simulink model "PTC_MBDS_SetBit_Sample"  (R2013a)
settings: Solver=FixedStepDiscrete  StartTime=0.0  StopTime=100  FixedStep=Auto  RelTol=1e-3
libraries: simulink x12, PTC_MBDS_LIB x4, simulink_extras x1
settings Model: Creator=uidl7367  LastModifiedBy=sundeep.tuteja
settings DataIOCC: SignalLoggingSaveFormat=ModelDataLogs
settings OptimizationCC: ExpressionDepthLimit=2147483647  InitFltsAndDblsToZero=on
settings DebuggingCC: SaveWithParameterizedLinksMsg=none  SignalResolutionControl=TryResolveAllWithWarning  SolverPrmCheckMsg=none  InheritedTsInSrcMsg=none  MultiTaskDSMMsg=warning  MultiTaskCondExecSysMsg=none  FcnCallInpInsideContextMsg=UseLocalSettings  StrictBusMsg=Warning
settings RTWCC: IncludeERTFirstTime=on
settings GRTTargetCC: TargetFcnLib=ansi_tfl_tmw.mat  CombineOutputUpdateFcns=off  GRTInterface=on

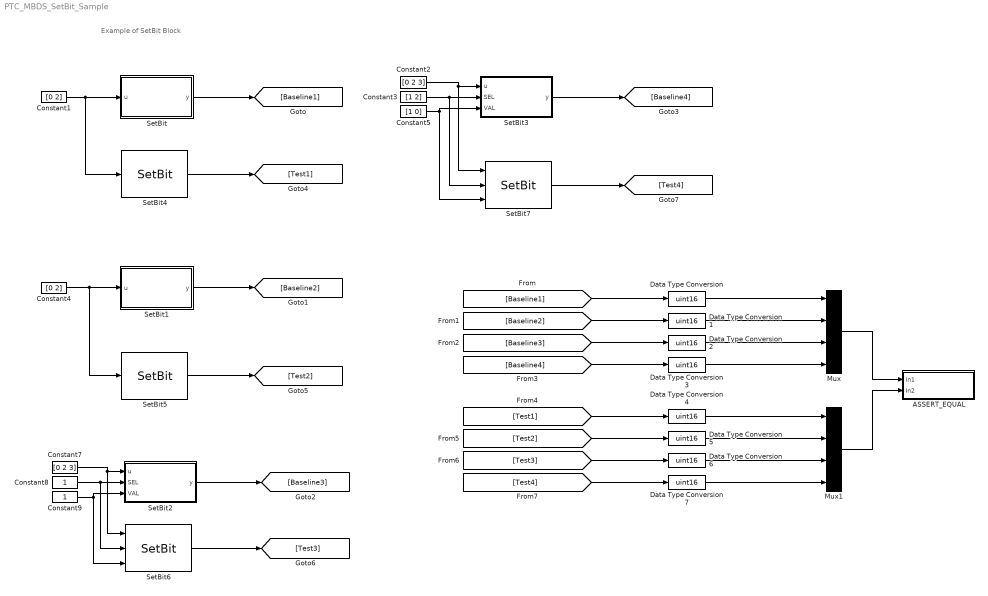
== system PTC_MBDS_SetBit_Sample ==
  note: Example of SetBit Block
  ASSERT_EQUAL : Subsystem
  Constant1 : Constant  InitFcn=|  Value=[0 2]  VectorParams1D=off  OutDataTypeStr=uint8
      | if(exist('MBDS_BlockCallback', 'file'))
      |    MBDS_BlockCallback('Update', gcb);  
      | end
  Constant2 : Constant  InitFcn=|  Value=[0 2 3]  VectorParams1D=off  OutDataTypeStr=uint16
      | if(exist('MBDS_BlockCallback', 'file'))
      |    MBDS_BlockCallback('Update', gcb);  
      | end
  Constant3 : Constant  InitFcn=|  Value=[1 2]  VectorParams1D=off  OutDataTypeStr=uint8
      | if(exist('MBDS_BlockCallback', 'file'))
      |    MBDS_BlockCallback('Update', gcb);  
      | end
  Constant4 : Constant  InitFcn=|  Value=[0 2]  VectorParams1D=off  OutDataTypeStr=uint8
      | if(exist('MBDS_BlockCallback', 'file'))
      |    MBDS_BlockCallback('Update', gcb);  
      | end
  Constant5 : Constant  InitFcn=|  Value=[1 0]  VectorParams1D=off  OutDataTypeStr=boolean
      | if(exist('MBDS_BlockCallback', 'file'))
      |    MBDS_BlockCallback('Update', gcb);  
      | end
  Constant7 : Constant  InitFcn=|  Value=[0 2 3]  VectorParams1D=off  OutDataTypeStr=uint16
      | if(exist('MBDS_BlockCallback', 'file'))
      |    MBDS_BlockCallback('Update', gcb);  
      | end
  Constant8 : Constant  InitFcn=|  VectorParams1D=off  OutDataTypeStr=uint8
      | if(exist('MBDS_BlockCallback', 'file'))
      |    MBDS_BlockCallback('Update', gcb);  
      | end
  Constant9 : Constant  InitFcn=|  VectorParams1D=off  OutDataTypeStr=boolean
      | if(exist('MBDS_BlockCallback', 'file'))
      |    MBDS_BlockCallback('Update', gcb);  
      | end
  Data Type Conversion{,1..7} (8 alike) : DataTypeConversion  OutDataTypeStr=uint16
  Mux : Mux
  Mux1 : Mux
  SetBit : Subsystem  InitFcn=|  mask(SetBit){MBDS_LibraryBlock=on, ZeroIndexing=off, SEL_Enabled=off, SEL=1, VAL_Enabled=off, VAL=1, MBDS_BlockVersion=05.40}
      | if(exist('MBDS_BlockCallback', 'file'))
      |    MBDS_BlockCallback('Update', gcb);
      | end
      mask prompts: MBDS_LibraryBlock "MBDS library block"; ZeroIndexing "Use zero-based indexing"; SEL_Enabled "Show SEL port"; SEL "Bit selection:"; VAL_Enabled "Show VAL port"; VAL "Bit value:"; MBDS_BlockVersion "Block version:"
      mask help: Set or reset specified bits of a input signal.
      mask init:
      | if(exist('MBDS_BlockCallback', 'file'))
      |    MBDS_BlockCallback('Init', gcb);
      | else
      |    % Disable all mask parameters
      |    MaskEnables = get_param(gcb, 'MaskEnables');
      |    for k = [1:length(MaskEnables)]
      |       MaskEnables{k} = 'off';
      |    end
      |    if(~isequal(MaskEnables, get_param(gcb, 'MaskEnables')))
      |       set_param(gcb, 'MaskEnables', MaskEnables);
      |    end
      | end
      settings: AttributesFormatString=|
      | Zero-based indexing: %<ZeroIndexing>
      | VAL = %<VAL>
      mask Help: eval(['open([workdir(''library_dir:''),''\Blockset\help\'',get_param(gcb,''MaskType''),''.html''])'])
      mask Callback ZeroIndexing:
      | % Adopt Value
      | if(exist('MBDS_BlockCallback', 'file'))
      |    MBDS_BlockCallback('ZeroIndexing', gcb);
      | end
      mask Callback SEL_Enabled:
      | % Update mask parameter dialog
      | if(exist('MBDS_BlockCallback', 'file'))
      |    MBDS_BlockCallback('SEL_Enabled', gcb);
      | end
      mask Callback SEL:
      | % Adopt Value
      | if(exist('MBDS_BlockCallback', 'file'))
      |    MBDS_BlockCallback('SEL', gcb);
      | end
      mask Callback VAL_Enabled:
      | % Update mask parameter dialog
      | if(exist('MBDS_BlockCallback', 'file'))
      |    MBDS_BlockCallback('VAL_Enabled', gcb);
      | end
      mask Callback VAL:
      | % Adopt Value
      | if(exist('MBDS_BlockCallback', 'file'))
      |    MBDS_BlockCallback('VAL', gcb);
      | end
      mask Display:
      | % Show block text
      | disp(sprintf('Set Bit'));
      | 
      | % Display port labels
      | port_label('input', 1, 'u');
      | port_label('output', 1, 'y');
  SetBit1 : Subsystem  InitFcn=|  mask(SetBit){MBDS_LibraryBlock=on, ZeroIndexing=on, SEL_Enabled=off, SEL=0, VAL_Enabled=off, VAL=1, MBDS_BlockVersion=05.40}
      | if(exist('MBDS_BlockCallback', 'file'))
      |    MBDS_BlockCallback('Update', gcb);
      | end
      mask prompts: MBDS_LibraryBlock "MBDS library block"; ZeroIndexing "Use zero-based indexing"; SEL_Enabled "Show SEL port"; SEL "Bit selection:"; VAL_Enabled "Show VAL port"; VAL "Bit value:"; MBDS_BlockVersion "Block version:"
      mask help: Set or reset specified bits of a input signal.
      mask init: same as PTC_MBDS_SetBit_Sample/SetBit
      settings: AttributesFormatString=|
      | Zero-based indexing: %<ZeroIndexing>
      | VAL = %<VAL>
      mask Help: eval(['open([workdir(''library_dir:''),''\Blockset\help\'',get_param(gcb,''MaskType''),''.html''])'])
      mask Callback ZeroIndexing:
      | % Adopt Value
      | if(exist('MBDS_BlockCallback', 'file'))
      |    MBDS_BlockCallback('ZeroIndexing', gcb);
      | end
      mask Callback SEL_Enabled:
      | % Update mask parameter dialog
      | if(exist('MBDS_BlockCallback', 'file'))
      |    MBDS_BlockCallback('SEL_Enabled', gcb);
      | end
      mask Callback SEL:
      | % Adopt Value
      | if(exist('MBDS_BlockCallback', 'file'))
      |    MBDS_BlockCallback('SEL', gcb);
      | end
      mask Callback VAL_Enabled:
      | % Update mask parameter dialog
      | if(exist('MBDS_BlockCallback', 'file'))
      |    MBDS_BlockCallback('VAL_Enabled', gcb);
      | end
      mask Callback VAL:
      | % Adopt Value
      | if(exist('MBDS_BlockCallback', 'file'))
      |    MBDS_BlockCallback('VAL', gcb);
      | end
      mask Display:
      | % Show block text
      | disp(sprintf('Set Bit'));
      | 
      | % Display port labels
      | port_label('input', 1, 'u');
      | port_label('output', 1, 'y');
  SetBit2 : Subsystem  InitFcn=|  mask(SetBit){MBDS_LibraryBlock=on, ZeroIndexing=off, SEL_Enabled=on, SEL=0, VAL_Enabled=on, VAL=0, MBDS_BlockVersion=05.40}
      | if(exist('MBDS_BlockCallback', 'file'))
      |    MBDS_BlockCallback('Update', gcb);
      | end
      mask prompts: MBDS_LibraryBlock "MBDS library block"; ZeroIndexing "Use zero-based indexing"; SEL_Enabled "Show SEL port"; SEL "Bit selection:"; VAL_Enabled "Show VAL port"; VAL "Bit value:"; MBDS_BlockVersion "Block version:"
      mask help: Set or reset specified bits of a input signal.
      mask init: same as PTC_MBDS_SetBit_Sample/SetBit
      settings: AttributesFormatString=Zero-based indexing: %<ZeroIndexing>
      mask Help: eval(['open([workdir(''library_dir:''),''\Blockset\help\'',get_param(gcb,''MaskType''),''.html''])'])
      mask Callback ZeroIndexing:
      | % Adopt Value
      | if(exist('MBDS_BlockCallback', 'file'))
      |    MBDS_BlockCallback('ZeroIndexing', gcb);
      | end
      mask Callback SEL_Enabled:
      | % Update mask parameter dialog
      | if(exist('MBDS_BlockCallback', 'file'))
      |    MBDS_BlockCallback('SEL_Enabled', gcb);
      | end
      mask Callback SEL:
      | % Adopt Value
      | if(exist('MBDS_BlockCallback', 'file'))
      |    MBDS_BlockCallback('SEL', gcb);
      | end
      mask Callback VAL_Enabled:
      | % Update mask parameter dialog
      | if(exist('MBDS_BlockCallback', 'file'))
      |    MBDS_BlockCallback('VAL_Enabled', gcb);
      | end
      mask Callback VAL:
      | % Adopt Value
      | if(exist('MBDS_BlockCallback', 'file'))
      |    MBDS_BlockCallback('VAL', gcb);
      | end
      mask Display:
      | % Show block text
      | disp(sprintf('Set Bit'));
      | 
      | % Display port labels
      | port_label('input', 1, 'u');
      | port_label('input', 2, 'SEL');
      | port_label('input', 3, 'VAL');
      | port_label('output', 1, 'y');
  SetBit3 : Subsystem  InitFcn=|  mask(SetBit){MBDS_LibraryBlock=on, ZeroIndexing=off, SEL_Enabled=on, SEL=0, VAL_Enabled=on, VAL=0, MBDS_BlockVersion=05.40}
      | if(exist('MBDS_BlockCallback', 'file'))
      |    MBDS_BlockCallback('Update', gcb);
      | end
      mask prompts: MBDS_LibraryBlock "MBDS library block"; ZeroIndexing "Use zero-based indexing"; SEL_Enabled "Show SEL port"; SEL "Bit selection:"; VAL_Enabled "Show VAL port"; VAL "Bit value:"; MBDS_BlockVersion "Block version:"
      mask help: Set or reset specified bits of a input signal.
      mask init: same as PTC_MBDS_SetBit_Sample/SetBit
      settings: AttributesFormatString=Zero-based indexing: %<ZeroIndexing>
      mask Help: eval(['open([workdir(''library_dir:''),''\Blockset\help\'',get_param(gcb,''MaskType''),''.html''])'])
      mask Callback ZeroIndexing:
      | % Adopt Value
      | if(exist('MBDS_BlockCallback', 'file'))
      |    MBDS_BlockCallback('ZeroIndexing', gcb);
      | end
      mask Callback SEL_Enabled:
      | % Update mask parameter dialog
      | if(exist('MBDS_BlockCallback', 'file'))
      |    MBDS_BlockCallback('SEL_Enabled', gcb);
      | end
      mask Callback SEL:
      | % Adopt Value
      | if(exist('MBDS_BlockCallback', 'file'))
      |    MBDS_BlockCallback('SEL', gcb);
      | end
      mask Callback VAL_Enabled:
      | % Update mask parameter dialog
      | if(exist('MBDS_BlockCallback', 'file'))
      |    MBDS_BlockCallback('VAL_Enabled', gcb);
      | end
      mask Callback VAL:
      | % Adopt Value
      | if(exist('MBDS_BlockCallback', 'file'))
      |    MBDS_BlockCallback('VAL', gcb);
      | end
      mask Display:
      | % Show block text
      | disp(sprintf('Set Bit'));
      | 
      | % Display port labels
      | port_label('input', 1, 'u');
      | port_label('input', 2, 'SEL');
      | port_label('input', 3, 'VAL');
      | port_label('output', 1, 'y');
  SetBit4 : PTC_MBDS_LIB/MBDS Standard Library/Basic Operations/Logic and Bit Operations/SetBit  ZeroIndexing=off  SEL_Enabled=off  SEL=1  VAL_Enabled=off  VAL=1  PTC_MBDS_BlockVersion=5.32  PTC_BlockType=PTC_MBDS_SetBit
      settings: AttributesFormatString=|
      | SEL = %<SEL>
      | VAL = %<VAL>
      | Zero-based indexing: %<ZeroIndexing>
  SetBit5 : PTC_MBDS_LIB/MBDS Standard Library/Basic Operations/Logic and Bit Operations/SetBit  ZeroIndexing=on  SEL_Enabled=off  SEL=0  VAL_Enabled=off  VAL=1  PTC_MBDS_BlockVersion=5.32  PTC_BlockType=PTC_MBDS_SetBit
      settings: AttributesFormatString=|
      | SEL = %<SEL>
      | VAL = %<VAL>
      | Zero-based indexing: %<ZeroIndexing>
  SetBit6 : PTC_MBDS_LIB/MBDS Standard Library/Basic Operations/Logic and Bit Operations/SetBit  ZeroIndexing=off  SEL_Enabled=on  SEL=0  VAL_Enabled=on  VAL=1  PTC_MBDS_BlockVersion=5.32  PTC_BlockType=PTC_MBDS_SetBit
      settings: AttributesFormatString=Zero-based indexing: %<ZeroIndexing>
  SetBit7 : PTC_MBDS_LIB/MBDS Standard Library/Basic Operations/Logic and Bit Operations/SetBit  ZeroIndexing=off  SEL_Enabled=on  SEL=0  VAL_Enabled=on  VAL=1  PTC_MBDS_BlockVersion=5.32  PTC_BlockType=PTC_MBDS_SetBit
      settings: AttributesFormatString=Zero-based indexing: %<ZeroIndexing>
  wires:
  Constant1/1 -> SetBit/1(u), SetBit4/1
  SetBit/1(y) -> [Baseline1]
  Constant4/1 -> SetBit1/1(u), SetBit5/1
  SetBit1/1(y) -> [Baseline2]
  Constant8/1 -> SetBit2/2(SEL), SetBit6/2
  SetBit2/1(y) -> [Baseline3]
  Constant2/1 -> SetBit3/1(u), SetBit7/1
  Constant3/1 -> SetBit3/2(SEL), SetBit7/2
  Constant5/1 -> SetBit3/3(VAL), SetBit7/3
  SetBit3/1(y) -> [Baseline4]
  Constant7/1 -> SetBit2/1(u), SetBit6/1
  Constant9/1 -> SetBit2/3(VAL), SetBit6/3
  SetBit4/1 -> [Test1]
  SetBit5/1 -> [Test2]
  SetBit6/1 -> [Test3]
  SetBit7/1 -> [Test4]
  [Baseline1] -> Data Type Conversion/1
  [Baseline2] -> Data Type Conversion1/1
  [Baseline4] -> Data Type Conversion3/1
  [Baseline3] -> Data Type Conversion2/1
  [Test3] -> Data Type Conversion6/1
  [Test4] -> Data Type Conversion7/1
  [Test2] -> Data Type Conversion5/1
  [Test1] -> Data Type Conversion4/1
  Mux/1 -> ASSERT_EQUAL/1(In1)
  Mux1/1 -> ASSERT_EQUAL/2(In2)
  Data Type Conversion/1 -> Mux/1
  Data Type Conversion1/1 -> Mux/2
  Data Type Conversion2/1 -> Mux/3
  Data Type Conversion3/1 -> Mux/4
  Data Type Conversion4/1 -> Mux1/1
  Data Type Conversion5/1 -> Mux1/2
  Data Type Conversion6/1 -> Mux1/3
  Data Type Conversion7/1 -> Mux1/4

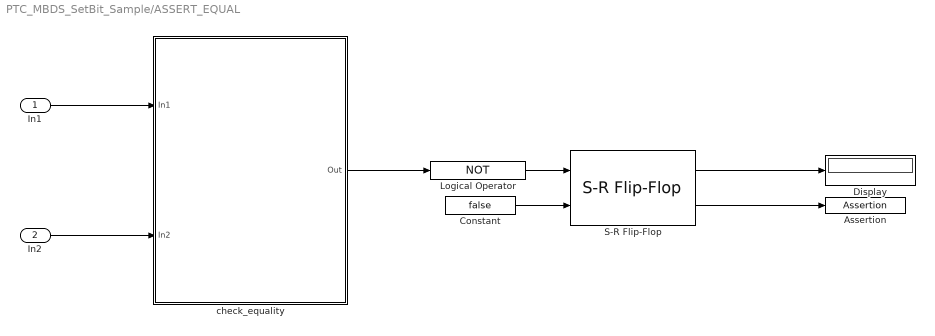
== system PTC_MBDS_SetBit_Sample/ASSERT_EQUAL ==
  In1 : Inport
  In2 : Inport  Port=2
  Assertion : Assertion
  Constant : Constant  Value=false
  Display : Display
  Logical Operator : Logic  Operator=NOT  AllPortsSameDT=off  OutDataTypeStr=boolean
  S-R Flip-Flop : simulink_extras/Flip Flops/S-R Flip-Flop  initial_condition=0
  check_equality : MATLAB Function  TreatAsAtomicUnit=on
  wires:
  S-R Flip-Flop/1 -> Display/1
  check_equality/1(Out) -> Logical Operator/1
  Constant/1 -> S-R Flip-Flop/2
  S-R Flip-Flop/2 -> Assertion/1
  In2/1 -> check_equality/2(In2)
  In1/1 -> check_equality/1(In1)
  Logical Operator/1 -> S-R Flip-Flop/1

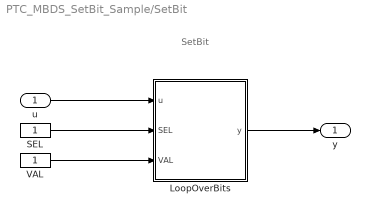
== system PTC_MBDS_SetBit_Sample/SetBit ==
  note: SetBit
  u : Inport
  LoopOverBits : Subsystem
  SEL : Constant  OutDataTypeStr=uint8
  VAL : Constant  OutDataTypeStr=boolean
  y : Outport
  wires:
  LoopOverBits/1(y) -> y/1
  VAL/1 -> LoopOverBits/3(VAL)
  SEL/1 -> LoopOverBits/2(SEL)
  u/1 -> LoopOverBits/1(u)

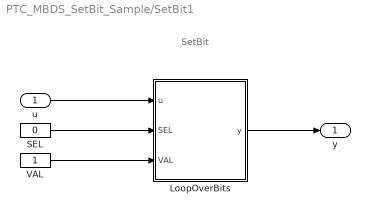
== system PTC_MBDS_SetBit_Sample/SetBit1 ==
  note: SetBit
  u : Inport
  LoopOverBits : Subsystem
  SEL : Constant  Value=0  OutDataTypeStr=uint8
  VAL : Constant  OutDataTypeStr=boolean
  y : Outport
  wires:
  LoopOverBits/1(y) -> y/1
  VAL/1 -> LoopOverBits/3(VAL)
  SEL/1 -> LoopOverBits/2(SEL)
  u/1 -> LoopOverBits/1(u)

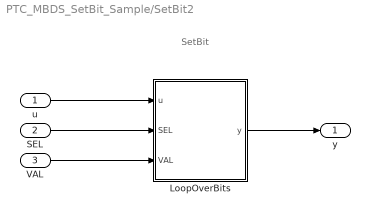
== system PTC_MBDS_SetBit_Sample/SetBit2 ==
  note: SetBit
  u : Inport
  SEL : Inport  Port=2
  VAL : Inport  Port=3  OutDataTypeStr=boolean
  LoopOverBits : Subsystem
  y : Outport
  wires:
  LoopOverBits/1(y) -> y/1
  VAL/1 -> LoopOverBits/3(VAL)
  SEL/1 -> LoopOverBits/2(SEL)
  u/1 -> LoopOverBits/1(u)

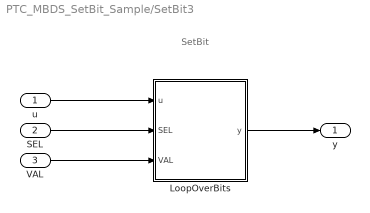
== system PTC_MBDS_SetBit_Sample/SetBit3 ==
  note: SetBit
  u : Inport
  SEL : Inport  Port=2
  VAL : Inport  Port=3  OutDataTypeStr=boolean
  LoopOverBits : Subsystem
  y : Outport
  wires:
  u/1 -> LoopOverBits/1(u)
  SEL/1 -> LoopOverBits/2(SEL)
  VAL/1 -> LoopOverBits/3(VAL)
  LoopOverBits/1(y) -> y/1

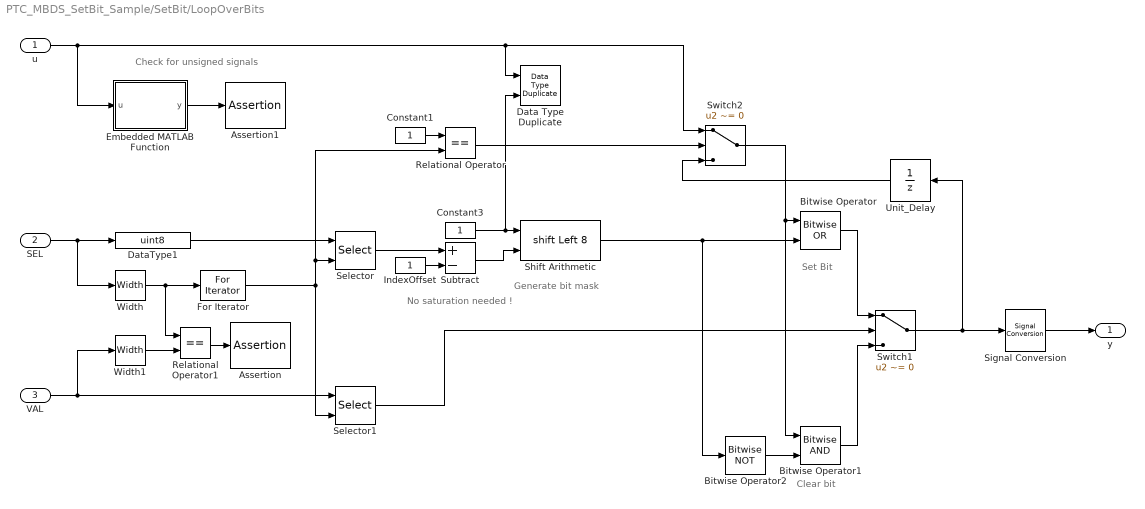
== system PTC_MBDS_SetBit_Sample/SetBit/LoopOverBits ==
  note: No saturation
      | needed !
  note: Generate bit mask
  note: Set Bit
  note: Clear bit
  note: Check for unsigned signals
  u : Inport
  SEL : Inport  Port=2
  VAL : Inport  Port=3
  Assertion : Assertion  AssertionFailFcn=error('Invalid signal dimensions. Bit selection and value specification should have the same dimensions.')
  Assertion1 : Assertion  AssertionFailFcn=error('Invalid data types used for set bit operation. Apply unsigned integer signals only.')
  Bitwise Operator : simulink/Logic and Bit Operations/Bitwise Operator  logicop=OR  UseBitMask=off  NumInputPorts=2  BitMask=bin2dec('11011001')  BitMaskRealWorld=Stored Integer
  Bitwise Operator1 : simulink/Logic and Bit Operations/Bitwise Operator  logicop=AND  UseBitMask=off  NumInputPorts=2  BitMask=bin2dec('11011001')  BitMaskRealWorld=Stored Integer
  Bitwise Operator2 : simulink/Logic and Bit Operations/Bitwise Operator  logicop=NOT  UseBitMask=off  BitMask=bin2dec('11011001')  BitMaskRealWorld=Stored Integer
  Constant1 : Constant  OutDataTypeStr=Inherit: Inherit via back propagation
  Constant3 : Constant  OutDataTypeStr=Inherit: Inherit via back propagation
  Data Type Duplicate : DataTypeDuplicate  InitFcn=|
      | try
      |    MBDS_BlockCallback('Update', gcb);
      | end
  DataType1 : DataTypeConversion  OutDataTypeStr=uint8
  Embedded MATLAB Function : MATLAB Function  TreatAsAtomicUnit=on
  For Iterator : ForIterator  IterationSource=external  IterationVariableDataType=int8
  IndexOffset : Constant  OutDataTypeStr=Inherit: Inherit via back propagation
  Relational Operator : RelationalOperator  Operator===  OutDataTypeStr=boolean
  Relational Operator1 : RelationalOperator  Operator===  OutDataTypeStr=boolean
  Selector : Selector  IndexOptions=Index vector (port)  Indices=[1 3]  OutputSizes=1
  Selector1 : Selector  IndexOptions=Index vector (port)  Indices=[1 3]  OutputSizes=1
  Shift Arithmetic : ArithShift  BitShiftNumberSource=Input port  BitShiftNumber=8  BitShiftDirection=Left
      settings: InputPortMap=u0,p1
  Signal Conversion : SignalConversion
  Subtract : Sum  Inputs=+-  OutDataTypeStr=Inherit: Inherit via back propagation  InputSameDT=on
  Switch1 : Switch  Criteria=u2 ~= 0
  Switch2 : Switch  Criteria=u2 ~= 0
  Unit_Delay : UnitDelay  InitFcn=|  SampleTime=-1
      | try                                  
      |    MBDS_BlockCallback('Update', gcb);
      | end
      settings: AttributesFormatString=Init = %<X0>
  Width : Width  DataType=uint8
  Width1 : Width  DataType=uint8
  y : Outport
  wires:
  Relational Operator1/1 -> Assertion/1
  Width1/1 -> Relational Operator1/2
  Relational Operator/1 -> Switch2/2
  Constant1/1 -> Relational Operator/1
  Unit_Delay/1 -> Switch2/3
  Switch2/1 -> Bitwise Operator1/1, Bitwise Operator/1
  For Iterator/1 -> Selector/2, Relational Operator/2, Selector1/2
  Width/1 -> Relational Operator1/1, For Iterator/1
  Selector1/1 -> Switch1/2
  Shift Arithmetic/1 -> Bitwise Operator2/1, Bitwise Operator/2
  Constant3/1 -> Data Type Duplicate/2, Shift Arithmetic/1
  Switch1/1 -> Signal Conversion/1, Unit_Delay/1
  Bitwise Operator/1 -> Switch1/1
  Bitwise Operator1/1 -> Switch1/3
  Bitwise Operator2/1 -> Bitwise Operator1/2
  Signal Conversion/1 -> y/1
  Subtract/1 -> Shift Arithmetic/2
  Selector/1 -> Subtract/1
  IndexOffset/1 -> Subtract/2
  SEL/1 -> DataType1/1, Width/1
  DataType1/1 -> Selector/1
  VAL/1 -> Selector1/1, Width1/1
  Embedded MATLAB Function/1(y) -> Assertion1/1
  u/1 -> Embedded MATLAB Function/1(u), Data Type Duplicate/1, Switch2/1

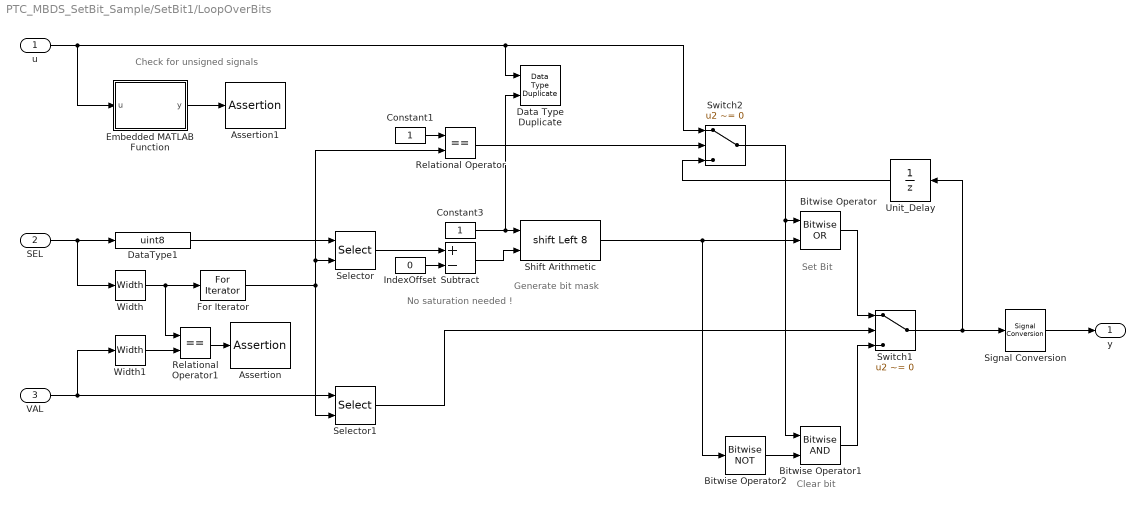
== system PTC_MBDS_SetBit_Sample/SetBit1/LoopOverBits ==
  note: No saturation
      | needed !
  note: Generate bit mask
  note: Set Bit
  note: Clear bit
  note: Check for unsigned signals
  u : Inport
  SEL : Inport  Port=2
  VAL : Inport  Port=3
  Assertion : Assertion  AssertionFailFcn=error('Invalid signal dimensions. Bit selection and value specification should have the same dimensions.')
  Assertion1 : Assertion  AssertionFailFcn=error('Invalid data types used for set bit operation. Apply unsigned integer signals only.')
  Bitwise Operator : simulink/Logic and Bit Operations/Bitwise Operator  logicop=OR  UseBitMask=off  NumInputPorts=2  BitMask=bin2dec('11011001')  BitMaskRealWorld=Stored Integer
  Bitwise Operator1 : simulink/Logic and Bit Operations/Bitwise Operator  logicop=AND  UseBitMask=off  NumInputPorts=2  BitMask=bin2dec('11011001')  BitMaskRealWorld=Stored Integer
  Bitwise Operator2 : simulink/Logic and Bit Operations/Bitwise Operator  logicop=NOT  UseBitMask=off  BitMask=bin2dec('11011001')  BitMaskRealWorld=Stored Integer
  Constant1 : Constant  OutDataTypeStr=Inherit: Inherit via back propagation
  Constant3 : Constant  OutDataTypeStr=Inherit: Inherit via back propagation
  Data Type Duplicate : DataTypeDuplicate  InitFcn=|
      | try
      |    MBDS_BlockCallback('Update', gcb);
      | end
  DataType1 : DataTypeConversion  OutDataTypeStr=uint8
  Embedded MATLAB Function : MATLAB Function  TreatAsAtomicUnit=on
  For Iterator : ForIterator  IterationSource=external  IterationVariableDataType=int8
  IndexOffset : Constant  Value=0  OutDataTypeStr=Inherit: Inherit via back propagation
  Relational Operator : RelationalOperator  Operator===  OutDataTypeStr=boolean
  Relational Operator1 : RelationalOperator  Operator===  OutDataTypeStr=boolean
  Selector : Selector  IndexOptions=Index vector (port)  Indices=[1 3]  OutputSizes=1
  Selector1 : Selector  IndexOptions=Index vector (port)  Indices=[1 3]  OutputSizes=1
  Shift Arithmetic : ArithShift  BitShiftNumberSource=Input port  BitShiftNumber=8  BitShiftDirection=Left
      settings: InputPortMap=u0,p1
  Signal Conversion : SignalConversion
  Subtract : Sum  Inputs=+-  OutDataTypeStr=Inherit: Inherit via back propagation  InputSameDT=on
  Switch1 : Switch  Criteria=u2 ~= 0
  Switch2 : Switch  Criteria=u2 ~= 0
  Unit_Delay : UnitDelay  InitFcn=|  SampleTime=-1
      | try                                  
      |    MBDS_BlockCallback('Update', gcb);
      | end
      settings: AttributesFormatString=Init = %<X0>
  Width : Width  DataType=uint8
  Width1 : Width  DataType=uint8
  y : Outport
  wires:
  Relational Operator1/1 -> Assertion/1
  Width1/1 -> Relational Operator1/2
  Relational Operator/1 -> Switch2/2
  Constant1/1 -> Relational Operator/1
  Unit_Delay/1 -> Switch2/3
  Switch2/1 -> Bitwise Operator1/1, Bitwise Operator/1
  For Iterator/1 -> Selector/2, Relational Operator/2, Selector1/2
  Width/1 -> Relational Operator1/1, For Iterator/1
  Selector1/1 -> Switch1/2
  Shift Arithmetic/1 -> Bitwise Operator2/1, Bitwise Operator/2
  Constant3/1 -> Data Type Duplicate/2, Shift Arithmetic/1
  Switch1/1 -> Signal Conversion/1, Unit_Delay/1
  Bitwise Operator/1 -> Switch1/1
  Bitwise Operator1/1 -> Switch1/3
  Bitwise Operator2/1 -> Bitwise Operator1/2
  Signal Conversion/1 -> y/1
  Subtract/1 -> Shift Arithmetic/2
  Selector/1 -> Subtract/1
  IndexOffset/1 -> Subtract/2
  SEL/1 -> DataType1/1, Width/1
  DataType1/1 -> Selector/1
  VAL/1 -> Selector1/1, Width1/1
  Embedded MATLAB Function/1(y) -> Assertion1/1
  u/1 -> Embedded MATLAB Function/1(u), Data Type Duplicate/1, Switch2/1

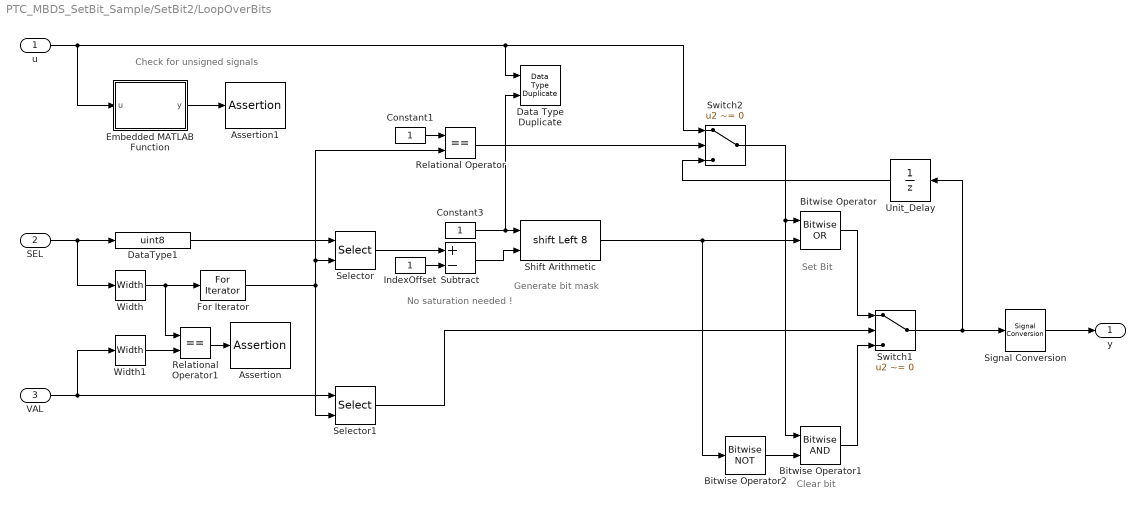
== system PTC_MBDS_SetBit_Sample/SetBit2/LoopOverBits ==
  note: No saturation
      | needed !
  note: Generate bit mask
  note: Set Bit
  note: Clear bit
  note: Check for unsigned signals
  u : Inport
  SEL : Inport  Port=2
  VAL : Inport  Port=3
  Assertion : Assertion  AssertionFailFcn=error('Invalid signal dimensions. Bit selection and value specification should have the same dimensions.')
  Assertion1 : Assertion  AssertionFailFcn=error('Invalid data types used for set bit operation. Apply unsigned integer signals only.')
  Bitwise Operator : simulink/Logic and Bit Operations/Bitwise Operator  logicop=OR  UseBitMask=off  NumInputPorts=2  BitMask=bin2dec('11011001')  BitMaskRealWorld=Stored Integer
  Bitwise Operator1 : simulink/Logic and Bit Operations/Bitwise Operator  logicop=AND  UseBitMask=off  NumInputPorts=2  BitMask=bin2dec('11011001')  BitMaskRealWorld=Stored Integer
  Bitwise Operator2 : simulink/Logic and Bit Operations/Bitwise Operator  logicop=NOT  UseBitMask=off  BitMask=bin2dec('11011001')  BitMaskRealWorld=Stored Integer
  Constant1 : Constant  OutDataTypeStr=Inherit: Inherit via back propagation
  Constant3 : Constant  OutDataTypeStr=Inherit: Inherit via back propagation
  Data Type Duplicate : DataTypeDuplicate  InitFcn=|
      | try
      |    MBDS_BlockCallback('Update', gcb);
      | end
  DataType1 : DataTypeConversion  OutDataTypeStr=uint8
  Embedded MATLAB Function : MATLAB Function  TreatAsAtomicUnit=on
  For Iterator : ForIterator  IterationSource=external  IterationVariableDataType=int8
  IndexOffset : Constant  OutDataTypeStr=Inherit: Inherit via back propagation
  Relational Operator : RelationalOperator  Operator===  OutDataTypeStr=boolean
  Relational Operator1 : RelationalOperator  Operator===  OutDataTypeStr=boolean
  Selector : Selector  IndexOptions=Index vector (port)  Indices=[1 3]  OutputSizes=1
  Selector1 : Selector  IndexOptions=Index vector (port)  Indices=[1 3]  OutputSizes=1
  Shift Arithmetic : ArithShift  BitShiftNumberSource=Input port  BitShiftNumber=8  BitShiftDirection=Left
      settings: InputPortMap=u0,p1
  Signal Conversion : SignalConversion
  Subtract : Sum  Inputs=+-  OutDataTypeStr=Inherit: Inherit via back propagation  InputSameDT=on
  Switch1 : Switch  Criteria=u2 ~= 0
  Switch2 : Switch  Criteria=u2 ~= 0
  Unit_Delay : UnitDelay  InitFcn=|  SampleTime=-1
      | try                                  
      |    MBDS_BlockCallback('Update', gcb);
      | end
      settings: AttributesFormatString=Init = %<X0>
  Width : Width  DataType=uint8
  Width1 : Width  DataType=uint8
  y : Outport
  wires:
  Relational Operator1/1 -> Assertion/1
  Width1/1 -> Relational Operator1/2
  Relational Operator/1 -> Switch2/2
  Constant1/1 -> Relational Operator/1
  Unit_Delay/1 -> Switch2/3
  Switch2/1 -> Bitwise Operator1/1, Bitwise Operator/1
  For Iterator/1 -> Selector/2, Relational Operator/2, Selector1/2
  Width/1 -> Relational Operator1/1, For Iterator/1
  Selector1/1 -> Switch1/2
  Shift Arithmetic/1 -> Bitwise Operator2/1, Bitwise Operator/2
  Constant3/1 -> Data Type Duplicate/2, Shift Arithmetic/1
  Switch1/1 -> Signal Conversion/1, Unit_Delay/1
  Bitwise Operator/1 -> Switch1/1
  Bitwise Operator1/1 -> Switch1/3
  Bitwise Operator2/1 -> Bitwise Operator1/2
  Signal Conversion/1 -> y/1
  Subtract/1 -> Shift Arithmetic/2
  Selector/1 -> Subtract/1
  IndexOffset/1 -> Subtract/2
  SEL/1 -> DataType1/1, Width/1
  DataType1/1 -> Selector/1
  VAL/1 -> Selector1/1, Width1/1
  Embedded MATLAB Function/1(y) -> Assertion1/1
  u/1 -> Embedded MATLAB Function/1(u), Data Type Duplicate/1, Switch2/1

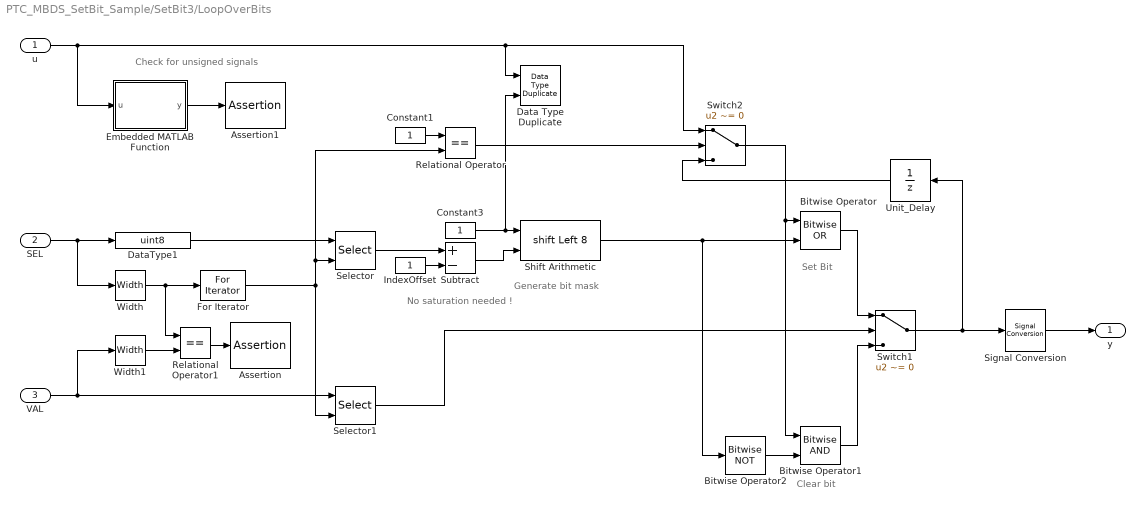
== system PTC_MBDS_SetBit_Sample/SetBit3/LoopOverBits ==
  note: Check for unsigned signals
  note: Clear bit
  note: Set Bit
  note: Generate bit mask
  note: No saturation
      | needed !
  u : Inport
  SEL : Inport  Port=2
  VAL : Inport  Port=3
  Assertion : Assertion  AssertionFailFcn=error('Invalid signal dimensions. Bit selection and value specification should have the same dimensions.')
  Assertion1 : Assertion  AssertionFailFcn=error('Invalid data types used for set bit operation. Apply unsigned integer signals only.')
  Bitwise Operator : simulink/Logic and Bit Operations/Bitwise Operator  logicop=OR  UseBitMask=off  NumInputPorts=2  BitMask=bin2dec('11011001')  BitMaskRealWorld=Stored Integer
  Bitwise Operator1 : simulink/Logic and Bit Operations/Bitwise Operator  logicop=AND  UseBitMask=off  NumInputPorts=2  BitMask=bin2dec('11011001')  BitMaskRealWorld=Stored Integer
  Bitwise Operator2 : simulink/Logic and Bit Operations/Bitwise Operator  logicop=NOT  UseBitMask=off  BitMask=bin2dec('11011001')  BitMaskRealWorld=Stored Integer
  Constant1 : Constant  OutDataTypeStr=Inherit: Inherit via back propagation
  Constant3 : Constant  OutDataTypeStr=Inherit: Inherit via back propagation
  Data Type Duplicate : DataTypeDuplicate  InitFcn=|
      | try
      |    MBDS_BlockCallback('Update', gcb);
      | end
  DataType1 : DataTypeConversion  OutDataTypeStr=uint8
  Embedded MATLAB Function : MATLAB Function  TreatAsAtomicUnit=on
  For Iterator : ForIterator  IterationSource=external  IterationVariableDataType=int8
  IndexOffset : Constant  OutDataTypeStr=Inherit: Inherit via back propagation
  Relational Operator : RelationalOperator  Operator===  OutDataTypeStr=boolean
  Relational Operator1 : RelationalOperator  Operator===  OutDataTypeStr=boolean
  Selector : Selector  IndexOptions=Index vector (port)  Indices=[1 3]  OutputSizes=1
  Selector1 : Selector  IndexOptions=Index vector (port)  Indices=[1 3]  OutputSizes=1
  Shift Arithmetic : ArithShift  BitShiftNumberSource=Input port  BitShiftNumber=8  BitShiftDirection=Left
      settings: InputPortMap=u0,p1
  Signal Conversion : SignalConversion
  Subtract : Sum  Inputs=+-  OutDataTypeStr=Inherit: Inherit via back propagation  InputSameDT=on
  Switch1 : Switch  Criteria=u2 ~= 0
  Switch2 : Switch  Criteria=u2 ~= 0
  Unit_Delay : UnitDelay  InitFcn=|  SampleTime=-1
      | try                                  
      |    MBDS_BlockCallback('Update', gcb);
      | end
      settings: AttributesFormatString=Init = %<X0>
  Width : Width  DataType=uint8
  Width1 : Width  DataType=uint8
  y : Outport
  wires:
  u/1 -> Switch2/1, Data Type Duplicate/1, Embedded MATLAB Function/1(u)
  Embedded MATLAB Function/1(y) -> Assertion1/1
  VAL/1 -> Width1/1, Selector1/1
  DataType1/1 -> Selector/1
  SEL/1 -> Width/1, DataType1/1
  IndexOffset/1 -> Subtract/2
  Selector/1 -> Subtract/1
  Subtract/1 -> Shift Arithmetic/2
  Signal Conversion/1 -> y/1
  Bitwise Operator2/1 -> Bitwise Operator1/2
  Bitwise Operator1/1 -> Switch1/3
  Bitwise Operator/1 -> Switch1/1
  Switch1/1 -> Unit_Delay/1, Signal Conversion/1
  Constant3/1 -> Shift Arithmetic/1, Data Type Duplicate/2
  Shift Arithmetic/1 -> Bitwise Operator/2, Bitwise Operator2/1
  Selector1/1 -> Switch1/2
  Width/1 -> For Iterator/1, Relational Operator1/1
  For Iterator/1 -> Selector1/2, Relational Operator/2, Selector/2
  Switch2/1 -> Bitwise Operator/1, Bitwise Operator1/1
  Unit_Delay/1 -> Switch2/3
  Constant1/1 -> Relational Operator/1
  Relational Operator/1 -> Switch2/2
  Width1/1 -> Relational Operator1/2
  Relational Operator1/1 -> Assertion/1

== matlab function PTC_MBDS_SetBit_Sample/SetBit/LoopOverBits/Embedded MATLAB Function ==
  data: u input; y output
function y = CheckType(u)

% Check for unsigned data types
if(isa(u,'uint8') || isa(u,'uint16') || isa(u,'uint32'))
   y = true;
else   
   y = false;
end

== matlab function PTC_MBDS_SetBit_Sample/SetBit1/LoopOverBits/Embedded MATLAB Function ==
  data: u input; y output
function y = CheckType(u)

% Check for unsigned data types
if(isa(u,'uint8') || isa(u,'uint16') || isa(u,'uint32'))
   y = true;
else   
   y = false;
end

== matlab function PTC_MBDS_SetBit_Sample/SetBit2/LoopOverBits/Embedded MATLAB Function ==
  data: u input; y output
function y = CheckType(u)

% Check for unsigned data types
if(isa(u,'uint8') || isa(u,'uint16') || isa(u,'uint32'))
   y = true;
else   
   y = false;
end

== matlab function PTC_MBDS_SetBit_Sample/SetBit3/LoopOverBits/Embedded MATLAB Function ==
  data: u input; y output
function y = CheckType(u)

% Check for unsigned data types
if(isa(u,'uint8') || isa(u,'uint16') || isa(u,'uint32'))
   y = true;
else   
   y = false;
end

== matlab function PTC_MBDS_SetBit_Sample/ASSERT_EQUAL/check_equality ==
  data: In1 input; Out output; In2 input
function Out = check_equality(In1, In2)
%#codegen

Out = isequaln(In1, In2);

end
